simulink model "simulacion_con_h"  (R2021a)
settings: Solver=VariableStepAuto  StartTime=0.0  StopTime=20  RelTol=1e-3
libraries: simulink x2
settings Model: Creator=franc  LastModifiedBy=facun

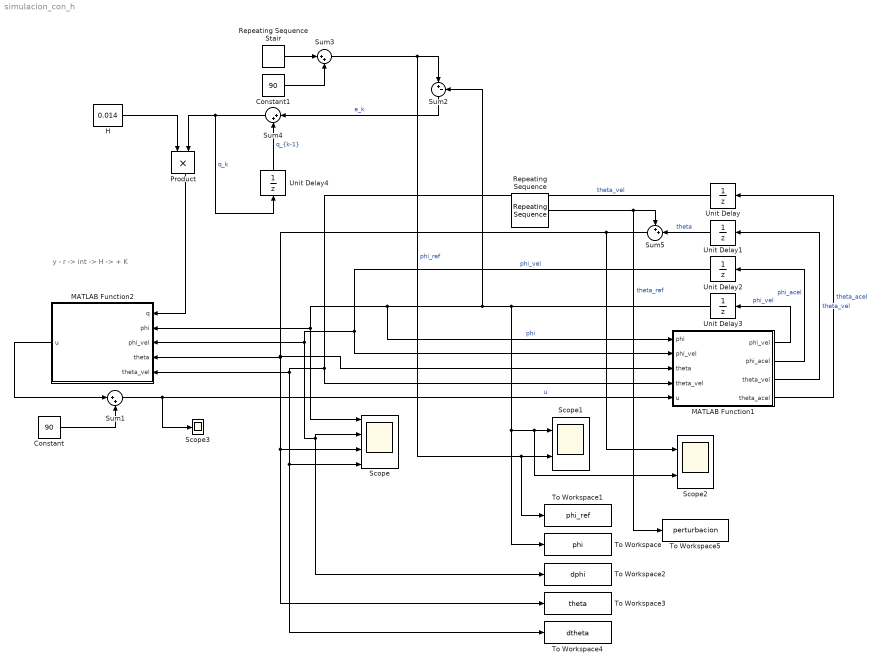
== system simulacion_con_h ==
  note: y - r -> int -> H -> + K
  Constant : Constant  Value=90
  Constant1 : Constant  Value=90
  H : Constant  Value=0.014
  MATLAB Function1 : MATLAB Function  TreatAsAtomicUnit=on
  MATLAB Function2 : MATLAB Function  TreatAsAtomicUnit=on
  Product : Product
  Repeating Sequence : simulink/Sources/Repeating Sequence  rep_seq_t=[0 0.01 0.10 0.18 4]  rep_seq_y=[0 0 5 0 0]
  Repeating Sequence Stair : simulink/Sources/Repeating Sequence Stair  OutValues=[0 0 0 0 0 0 0]  tsamp=6  OutMin=[]  OutMax=[]  OutDataTypeStr=double  OutputDataTypeScalingMode=double  OutDataType=fixdt(0,8)  ConRadixGroup=Best Precision: Vector-wise  OutScaling=2^-12
  Scope : Scope  NumInputPorts=4
  Scope1 : Scope  NumInputPorts=2
  Scope2 : Scope  NumInputPorts=2
  Scope3 : Scope
  Sum1 : Sum  Inputs=|++
  Sum2 : Sum  Inputs=|+-
  Sum3 : Sum  Inputs=|++
  Sum4 : Sum  Inputs=|++
  Sum5 : Sum  Inputs=++|
  To Workspace : ToWorkspace  VariableName=phi  SampleTime=-1
      settings: Save2DSignal=2-D array (concatenate along first dimension)
  To Workspace1 : ToWorkspace  VariableName=phi_ref  SampleTime=-1
      settings: Save2DSignal=2-D array (concatenate along first dimension)
  To Workspace2 : ToWorkspace  VariableName=dphi  SampleTime=-1
      settings: Save2DSignal=2-D array (concatenate along first dimension)
  To Workspace3 : ToWorkspace  VariableName=theta  SampleTime=-1
      settings: Save2DSignal=2-D array (concatenate along first dimension)
  To Workspace4 : ToWorkspace  VariableName=dtheta  SampleTime=-1
      settings: Save2DSignal=2-D array (concatenate along first dimension)
  To Workspace5 : ToWorkspace  VariableName=perturbacion  SampleTime=-1
      settings: Save2DSignal=2-D array (concatenate along first dimension)
  Unit Delay{,1..2,4} (4 alike) : UnitDelay  SampleTime=0.01  HasFrameUpgradeWarning=on
  Unit Delay3 : UnitDelay  InitialCondition=90  SampleTime=0.01  HasFrameUpgradeWarning=on
  wires:
  MATLAB Function1/1(phi_vel) -> Unit Delay3/1  "phi_vel"
  MATLAB Function1/2(phi_acel) -> Unit Delay2/1  "phi_acel"
  Unit Delay2/1 -> MATLAB Function2/3(phi_vel), To Workspace2/1, Scope/2, MATLAB Function1/2("phi_vel ")  "phi_vel"
  MATLAB Function1/3(theta_vel) -> Unit Delay1/1  "theta_vel"
  MATLAB Function1/4(theta_acel) -> Unit Delay/1  "theta_acel"
  Unit Delay3/1 -> To Workspace/1, Scope2/2, Scope1/1, MATLAB Function1/1(phi), Scope/1, MATLAB Function2/2(phi), Sum2/2  "phi"
  Sum1/1 -> Scope3/1, MATLAB Function1/5(u)  "u"
  Constant/1 -> Sum1/2
  Unit Delay/1 -> MATLAB Function1/4("theta_vel "), To Workspace4/1, Scope/4, MATLAB Function2/5(theta_vel)  "theta_vel"
  MATLAB Function2/1(u) -> Sum1/1
  Repeating Sequence Stair/1 -> Sum3/1
  Constant1/1 -> Sum3/2
  Sum3/1 -> To Workspace1/1, Scope1/2, Sum2/1  "phi_ref"
  Sum4/1 -> Product/2, Unit Delay4/1  "q_k"
  Product/1 -> MATLAB Function2/1(q)
  H/1 -> Product/1
  Sum2/1 -> Sum4/1  "e_k"
  Unit Delay4/1 -> Sum4/2  "q_{k-1}"
  Repeating Sequence/1 -> To Workspace5/1, Sum5/1  "theta_ref"
  Sum5/1 -> To Workspace3/1, Scope/3, MATLAB Function2/4(theta), MATLAB Function1/3(theta), Scope2/1
  Unit Delay1/1 -> Sum5/2  "theta"

== matlab function simulacion_con_h/MATLAB Function1 ==
  data: phi input; phi_vel input; theta input; theta_vel input; u input; phi_vel output; phi_acel output; theta_vel output; theta_acel output
function [phi_vel,phi_acel,theta_vel,theta_acel] = fcn(phi,phi_vel,theta,theta_vel,u)

Ad = [
    1.0000    0.0100         0         0;
   -0.5765    0.9895   -2.1322   -0.2132;
         0         0    1.0000    0.0100;
         0         0   -2.5000    0.7500;
];
   
Bd = [
         0;
  2.132250;
         0;
  2.500000
];

x  = [theta theta_vel phi phi_vel];
x_dot = Ad * x' + Bd * u;
theta_vel = x_dot(1);
theta_acel = x_dot(2);
phi_vel = x_dot(3);
phi_acel = x_dot(4);

== matlab function simulacion_con_h/MATLAB Function2 ==
  data: q input; phi input; phi_vel input; theta input; theta_vel input; u output
function u = fcn(q, phi,phi_vel,theta,theta_vel)
    K = [-0.5   0.05    0.3    -0.03]; % K integral
    u = K(1) * theta + K(2) * theta_vel + K(3) * (phi - 90) + K(4) * phi_vel + q;
